simulink model "Suspension"  (R2020a)
settings: Solver=VariableStepAuto  StartTime=0.0  StopTime=10.0  RelTol=1e-3
values from neighbouring files (symbols this model uses):
  Cf = 2500    [Suspension_Datas.m]
  Cr = 2000    [Suspension_Datas.m]
  Iyy = 2100    [Suspension_Datas.m]
  Kf = 1    [ABS_Datas.m]    (also in Suspension_Datas.m = 28000)
  Kr = 21000    [Suspension_Datas.m]
  Lf = 0.9    [Suspension_Datas.m]
  Lr = 1.2    [Suspension_Datas.m]
  mb = 1200    [Suspension_Datas.m]
settings Model: Creator=Yogesh  LastModifiedBy=guru2

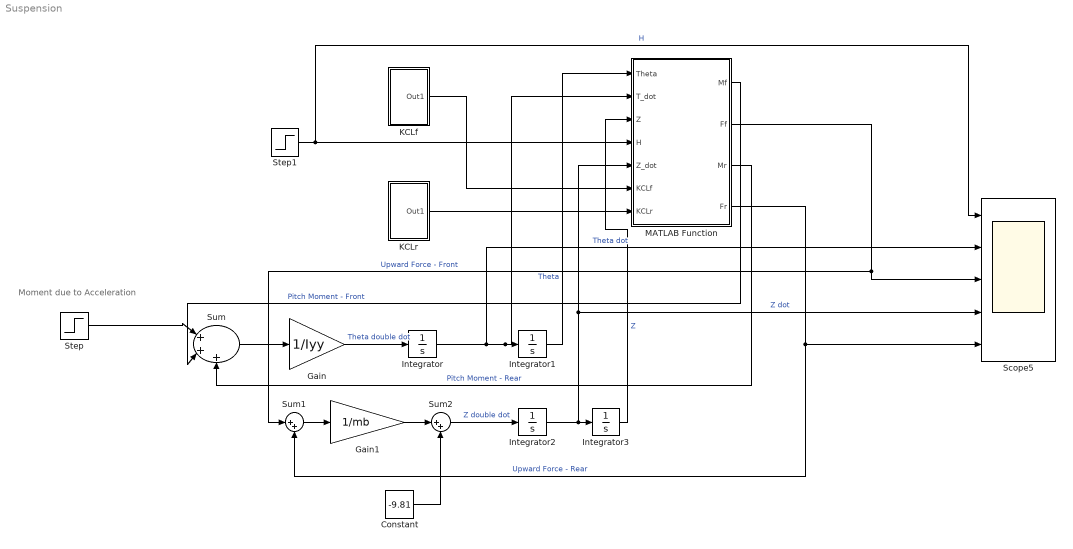
== system Suspension ==
  note: Moment due to Acceleration
  Constant : Constant  Value=-9.81
  Gain : Gain  Gain=1/Iyy
  Gain1 : Gain  Gain=1/mb
  Integrator{,1..3} (4 alike) : Integrator
  KCLf : Subsystem
  KCLr : Subsystem
  MATLAB Function : MATLAB Function  TreatAsAtomicUnit=on
  Scope5 : Scope  NumInputPorts=5
  Step : Step  Time=3  After=1000  SampleTime=0
  Step1 : Step  Time=7  After=5  SampleTime=0
  Sum : Sum  Inputs=|+++
  Sum1 : Sum  Inputs=|++
  Sum2 : Sum  Inputs=|++
  wires:
  Step/1 -> Sum/1
  Sum/1 -> Gain/1
  Gain/1 -> Integrator/1  "Theta double dot"
  Integrator/1 -> MATLAB Function/2(T_dot), Integrator1/1, Scope5/2  "Theta dot"
  Integrator1/1 -> MATLAB Function/1(Theta)  "Theta"
  Sum1/1 -> Gain1/1
  Gain1/1 -> Sum2/1
  Sum2/1 -> Integrator2/1  "Z double dot"
  Integrator2/1 -> Integrator3/1, MATLAB Function/5(Z_dot), Scope5/4  "Z dot"
  Integrator3/1 -> MATLAB Function/3(Z)  "Z"
  Step1/1 -> Scope5/1, MATLAB Function/4(H)  "H"
  Constant/1 -> Sum2/2
  KCLf/1(Out1) -> MATLAB Function/6(KCLf)
  KCLr/1(Out1) -> MATLAB Function/7(KCLr)
  MATLAB Function/3(Mr) -> Sum/3  "Pitch Moment - Rear"
  MATLAB Function/4(Fr) -> Sum1/2, Scope5/5  "Upward Force - Rear"
  MATLAB Function/2(Ff) -> Scope5/3, Sum1/1  "Upward Force - Front"
  MATLAB Function/1(Mf) -> Sum/2  "Pitch Moment - Front"

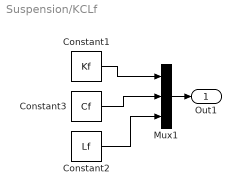
== system Suspension/KCLf ==
  Constant1 : Constant  Value=Kf
  Constant2 : Constant  Value=Lf
  Constant3 : Constant  Value=Cf
  Mux1 : Mux  Inputs=3
  Out1 : Outport
  wires:
  Constant1/1 -> Mux1/1
  Constant3/1 -> Mux1/2
  Constant2/1 -> Mux1/3
  Mux1/1 -> Out1/1

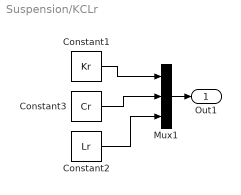
== system Suspension/KCLr ==
  Constant1 : Constant  Value=Kr
  Constant2 : Constant  Value=Lr
  Constant3 : Constant  Value=Cr
  Mux1 : Mux  Inputs=3
  Out1 : Outport
  wires:
  Mux1/1 -> Out1/1
  Constant2/1 -> Mux1/3
  Constant3/1 -> Mux1/2
  Constant1/1 -> Mux1/1

== matlab function Suspension/MATLAB Function ==
  data: Theta input; Mf output; T_dot input; Z input; H input; Z_dot input; KCLf input; KCLr input; Ff output; Mr output; Fr output
function [Mf,Ff,Mr,Fr] = fcn(Theta,T_dot,Z,H,Z_dot,KCLf,KCLr)
Kf = KCLf(1);   Cf = KCLf(2);   Lf = KCLf(3);
Kr = KCLr(1);   Cr = KCLr(2);   Lr = KCLr(3);
Ff = -2*Kf*(Z+H) + 2*Kf*Lf*Theta - 2*Cf*Z_dot + 2*Cf*Lf*T_dot;
Mf = -Ff*Lf;
Fr = -2*Kr*(Z+H) - 2*Kr*Lr*Theta - 2*Cr*Z_dot - 2*Cr*Lr*T_dot;
Mr = Fr*Lr;
